simulink model "Question12_AkankshaMurali"  (R2023b)
settings: Solver=VariableStepAuto  StartTime=0.0  StopTime=10.0  RelTol=1e-3
settings Model: Creator=akank  LastModifiedBy=akank

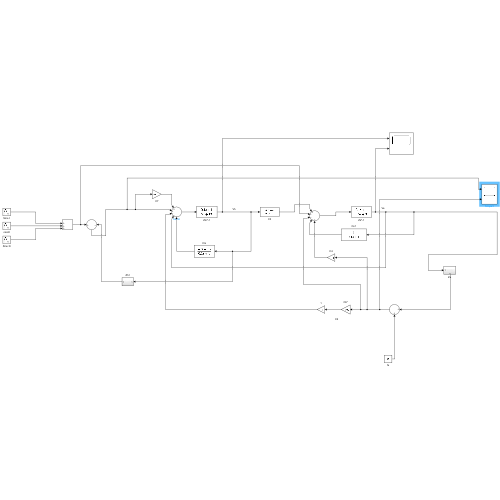
[thumbnail: Simulink's stored preview of the top-level diagram]
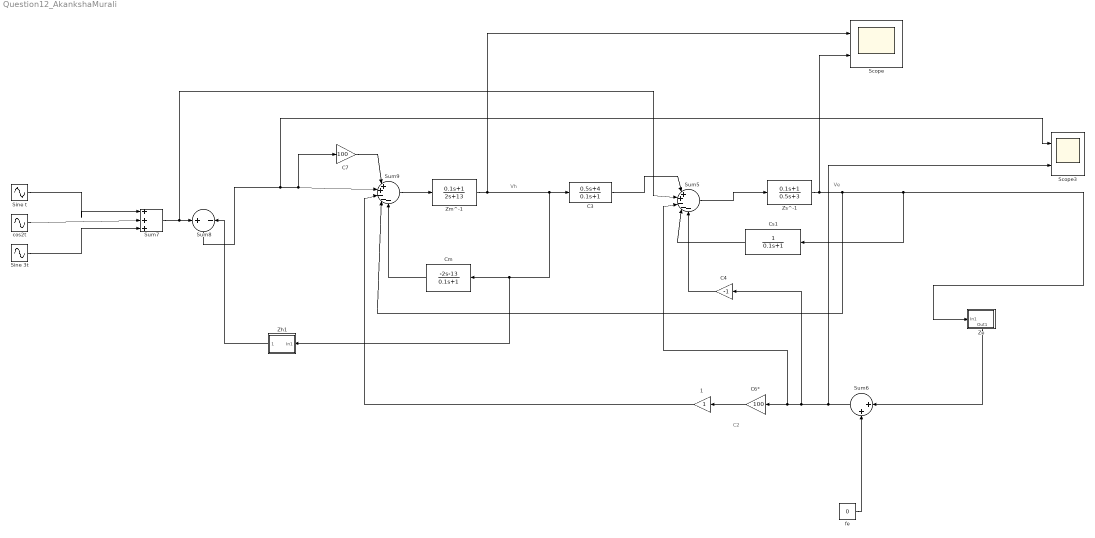
== system Question12_AkankshaMurali ==
  note: C2
  note: Ve
  note: Vh
  1 : Gain
  C3 : TransferFcn  Numerator=[0.5 4]  Denominator=[0.1 1]
  C4 : Gain  Gain=-1
  C6* : Gain  Gain=100
  C7 : Gain  Gain=100
  Cm : TransferFcn  Numerator=[-2 -13]  Denominator=[0.1 1]
  Cs1 : TransferFcn  Denominator=[0.1 1]
  Scope : Scope  NumInputPorts=2
  Scope3 : Scope  NumInputPorts=2
  Sine 3t : Sin  Frequency=3  SampleTime=0
  Sine t : Sin  SampleTime=0
  Sum5 : Sum  Inputs=|++---
  Sum6 : Sum  Inputs=|++
  Sum7 : Sum  Inputs=|+++
  Sum8 : Sum  Inputs=+-
  Sum9 : Sum  Inputs=|++---
  Ze : Subsystem
      settings: PortSchema="{\"entries\":[{\"content\":{\"sides\":[{\"content\":{\"connectorIds\":[\"In1\"]},\"type\":\"ConnectorPlacement.EquallySpacedRectSide\",\"uuid\":\"027018de-2e34-44dd-ab9f-8471e5e33890\"},{\"content\":{\"side\":\"RIGHT\"},\"type\":\"ConnectorPlacement.EquallySpacedRectSide\",\"uuid\":\"4715c82c-b0f0-4486-943a-5dc51080262b\"},{\"content\":{\"side\":\"TOP\"},\"type\":\"ConnectorPlacement.EquallySpacedRectSide\",\"uuid\":\"4872dab4-2133-4509-a71c-aeb9b0f2bdd1\"},{\"content\":{\"connectorIds\":[\"Out1\"],\"side\":\"BOTTOM\"},\"type\":\"ConnectorPlacement.EquallySpacedRectSide\",\"uuid\":\"b7f56b99-43be-41ae-a453-ea8486df40b4\"}]},\"type\":\"ConnectorPlacement.EquallySpacedConnector\",\"uuid\":\"3cfe3fcb-9aab-49ca-8c22-661775f2883d\"}],\"packageUris\":[\"http://schema.mathworks.com/mf0/Connector/R2020b\"],\"version\":\"1.0\"}"
  Zh1 : Subsystem
  Zm^-1 : TransferFcn  Numerator=[0.1 1]  Denominator=[2 13]
  Zs^-1 : TransferFcn  Numerator=[0.1 1]  Denominator=[0.5 3]
  cos2t : Sin  Frequency=2  Phase=pi/2  SampleTime=0
  fe : Constant  Value=0
  wires:
  1/1 -> Sum9/3
  fe/1 -> Sum6/2
  Cs1/1 -> Sum5/4
  Sum7/1 -> Sum5/2, Sum8/1
  C4/1 -> Sum5/5
  Sum6/1 -> C4/1, Sum5/3, C6*/1, Scope3/2
  Ze/1(Out1) -> Sum6/1
  Zm^-1/1 -> Scope/1, Zh1/1(In1), Cm/1, C3/1
  Sum8/1 -> Sum9/2, C7/1, Scope3/1
  C7/1 -> Sum9/1
  Zs^-1/1 -> Scope/2, Ze/1(In1), Cs1/1, Sum9/4
  Zh1/1(Out1) -> Sum8/2
  C6*/1 -> 1/1
  Sum9/1 -> Zm^-1/1
  cos2t/1 -> Sum7/2
  Sum5/1 -> Zs^-1/1
  C3/1 -> Sum5/1
  Sine 3t/1 -> Sum7/3
  Sine t/1 -> Sum7/1
  Cm/1 -> Sum9/5

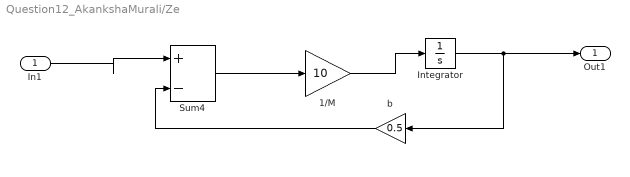
== system Question12_AkankshaMurali/Ze ==
  In1 : Inport
  1/M : Gain  Gain=10
  Integrator : Integrator  InitialCondition=2
  Sum4 : Sum  Inputs=|+-
  b : Gain  Gain=0.5
  Out1 : Outport
  wires:
  b/1 -> Sum4/2
  Sum4/1 -> 1/M/1
  In1/1 -> Sum4/1
  Integrator/1 -> Out1/1, b/1
  1/M/1 -> Integrator/1

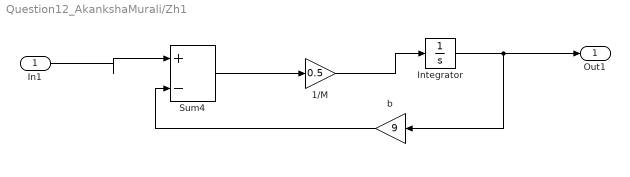
== system Question12_AkankshaMurali/Zh1 ==
  In1 : Inport
  1/M : Gain  Gain=0.5
  Integrator : Integrator  InitialCondition=2
  Sum4 : Sum  Inputs=|+-
  b : Gain  Gain=9
  Out1 : Outport
  wires:
  Integrator/1 -> Out1/1, b/1
  In1/1 -> Sum4/1
  b/1 -> Sum4/2
  Sum4/1 -> 1/M/1
  1/M/1 -> Integrator/1
